simulink model "mbed_disco_f407_encoder"  (R2015a)
settings: Solver=FixedStepDiscrete  SolverMode=SingleTasking  StartTime=0.0  StopTime=10.0  FixedStep=1e-3  RelTol=1e-3
libraries: mbed_targets_stm_disco_f407 x6, simulink x4
settings Model: Creator=oh  LastModifiedBy=oh
settings OptimizationCC: OptimizeModelRefInitCode=on  LifeSpan=1
settings HardwareCC: ProdLargestAtomicInteger=Long  ProdLargestAtomicFloat=Double  ProdEndianess=LittleEndian  ProdHWDeviceType=ARM Compatible->ARM Cortex
settings RTWCC: SystemTargetFile=mbed.tlc  TemplateMakefile=mbed.tmf  Description=Mbed Target (Embedded Target)  TargetLang=C++
settings CodeAppCC: IgnoreCustomStorageClasses=off
settings STFCustomTargetCC: CombineOutputUpdateFcns=on  SupportContinuousTime=off  SupportVariableSizeSignals=off  SystemTargetFile=mbed.tlc
settings ERTTargetCC: SupportContinuousTime=off  SupportVariableSizeSignals=off  ERTCustomFileTemplate=mbed_file_process.tlc

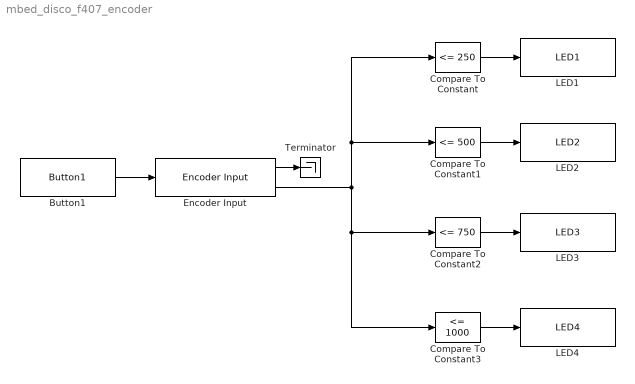
== system mbed_disco_f407_encoder ==
  Button1 : mbed_targets_stm_disco_f407/Button1  Parameter1=0
      link override Digital Input: SampleTime=1e-3
  Compare To Constant : simulink/Logic and Bit Operations/Compare To Constant  relop=<=  const=250  OutDataTypeStr=uint8
  Compare To Constant1 : simulink/Logic and Bit Operations/Compare To Constant  relop=<=  const=500  OutDataTypeStr=uint8
  Compare To Constant2 : simulink/Logic and Bit Operations/Compare To Constant  relop=<=  const=750  OutDataTypeStr=uint8
  Compare To Constant3 : simulink/Logic and Bit Operations/Compare To Constant  relop=<=  const=1000  OutDataTypeStr=uint8
  Encoder Input : mbed_targets_stm_disco_f407/Encoder Input  TimerNumber=TIM1  EncoderMode=TI1  Ti1Port=A  Ti1Pin=0  Ti2Port=A  Ti2Pin=0  InputMode=PullNone  Resolution=1000  SampleTime=-1
  LED1 : mbed_targets_stm_disco_f407/LED1  Parameter1=0
  LED2 : mbed_targets_stm_disco_f407/LED2  Parameter1=0
  LED3 : mbed_targets_stm_disco_f407/LED3  Parameter1=0
  LED4 : mbed_targets_stm_disco_f407/LED4  Parameter1=0
  Terminator : Terminator
  wires:
  Button1/1 -> Encoder Input/1
  Compare To Constant/1 -> LED1/1
  Encoder Input/2 -> Compare To Constant3/1, Compare To Constant2/1, Compare To Constant/1, Compare To Constant1/1
  Compare To Constant3/1 -> LED4/1
  Compare To Constant2/1 -> LED3/1
  Compare To Constant1/1 -> LED2/1
  Encoder Input/1 -> Terminator/1
